simulink model "ControlAllocator"  (R2025b)
settings: Solver=VariableStepAuto  StartTime=0.0  StopTime=10.0  RelTol=1e-3
settings Model: Creator=bohdanusatov  LastModifiedBy=bohdanusatov

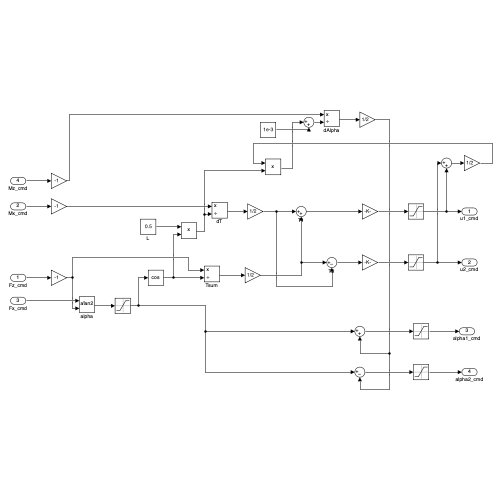
[thumbnail: Simulink's stored preview of the top-level diagram]
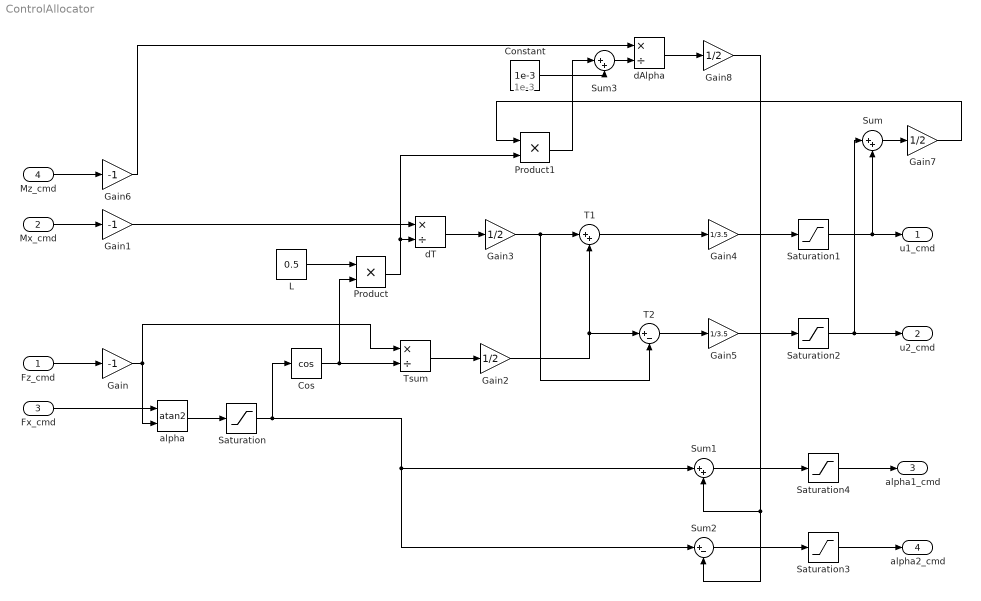
== system ControlAllocator ==
  note: 1e-3
  Fz_cmd : Inport
  Mx_cmd : Inport  Port=2
  Fx_cmd : Inport  Port=3
  Mz_cmd : Inport  Port=4
  Constant : Constant  Value=1e-3
  Cos : Trigonometry  Operator=cos
  Gain : Gain  Gain=-1
  Gain1 : Gain  Gain=-1
  Gain{2..3,7..8} (4 alike) : Gain  Gain=1/2
  Gain4 : Gain  Gain=1/3.5
  Gain5 : Gain  Gain=1/3.5
  Gain6 : Gain  Gain=-1
  L : Constant  Value=0.5
  Product : Product
  Product1 : Product
  Saturation : Saturate  UpperLimit=1  LowerLimit=-1
  Saturation1 : Saturate  UpperLimit=1  LowerLimit=0
  Saturation2 : Saturate  UpperLimit=1  LowerLimit=0
  Saturation3 : Saturate
  Saturation4 : Saturate
  Sum : Sum  Inputs=|++
  Sum1 : Sum  Inputs=|++
  Sum2 : Sum  Inputs=|+-
  Sum3 : Sum  Inputs=|++
  T1 : Sum  Inputs=|++
  T2 : Sum  Inputs=|+-
  Tsum : Product  Inputs=*/
  alpha : Trigonometry  Operator=atan2
  dAlpha : Product  Inputs=*/
  dT : Product  Inputs=*/
  u1_cmd : Outport
  u2_cmd : Outport  Port=2
  alpha1_cmd : Outport  Port=3
  alpha2_cmd : Outport  Port=4
  wires:
  Fx_cmd/1 -> alpha/1
  Fz_cmd/1 -> Gain/1
  Gain/1 -> alpha/2, Tsum/1
  alpha/1 -> Saturation/1
  Saturation/1 -> Cos/1, Sum2/1, Sum1/1
  Cos/1 -> Product/2, Tsum/2
  L/1 -> Product/1
  Mx_cmd/1 -> Gain1/1
  Product/1 -> Product1/2, dT/2
  Gain1/1 -> dT/1
  Tsum/1 -> Gain2/1
  dT/1 -> Gain3/1
  Gain3/1 -> T2/2, T1/1
  Gain2/1 -> T1/2, T2/1
  Saturation1/1 -> Sum/2, u1_cmd/1
  Saturation2/1 -> Sum/1, u2_cmd/1
  Gain5/1 -> Saturation2/1
  Gain4/1 -> Saturation1/1
  T1/1 -> Gain4/1
  T2/1 -> Gain5/1
  Mz_cmd/1 -> Gain6/1
  Sum/1 -> Gain7/1
  Gain7/1 -> Product1/1
  Gain6/1 -> dAlpha/1
  Product1/1 -> Sum3/1
  dAlpha/1 -> Gain8/1
  Gain8/1 -> Sum2/2, Sum1/2
  Sum1/1 -> Saturation4/1
  Sum2/1 -> Saturation3/1
  Saturation3/1 -> alpha2_cmd/1
  Saturation4/1 -> alpha1_cmd/1
  Constant/1 -> Sum3/2
  Sum3/1 -> dAlpha/2
